simulink model "rtlsdr_rx_combinetwo"  (R2014b)
settings: Solver=ode45  StartTime=0.0  StopTime=inf  RelTol=1e-3
PreLoadFcn:
  | %%%%%%%%%%%%%%%%%%%%%%%%%%%%%%%%%%%%%%%%%%%%%%%%%%%%%%%%%%%%%%%%%%%%%%%%%%%
  | % check to see if Simulink library folder is missing from the MATLAB path %
  | %%%%%%%%%%%%%%%%%%%%%%%%%%%%%%%%%%%%%%%%%%%%%%%%%%%%%%%%%%%%%%%%%%%%%%%%%%%
  | if isempty(strfind(path, 'rtlsdr_book_library'))
  | 
  |     % create error window
  |     fig_error = figure(...
  |         'Name', 'Error: RTL-SDR Book Library',...
  |         'Toolbar','none',...
  |         'MenuBar','none',...
  |         'NumberTitle','off',...
  |         'Resize','off',...
  |         'WindowStyle','modal');
  |     fig_error.Position(3) = 600;
  |     fig_error.Position(4) = 150;
  |     fig_axes = axes(...
  |         'Parent',fig_error,...
  |         'Position',[0,0,1,1],...
  |         'visible','off');
  |     % error message
  |     t_title = text(.05,.8,...
  |         'MISSING DIRECTORIES',...
  |         'FontSize',11.5);
  |     t_body = text(.075,.6,...
  |         [{'Simulink cannot find the  \it{<root>}\rm / \it{rtlsdr\_book\_library}\rm  folder in the \it{MATLAB Path}\rm.'},...
  |         {'Please set the MATLAB path following the instructions given in Exercise 2.4.'}],...
  |         'FontSize',10.5);
  |     % buttons
  |     btn_path = uicontrol(...
  |         'Parent',fig_error,...
  |         'String','Set Path Now',...
  |         'FontSize',10,...
  |         'Callback', 'pathtool; close(fig_error);',...
  |         'Position', [fig_error.Position(3)/2-210, 30, 200, 30]);
  |     btn_abort = uicontrol(...
  |         'Parent',fig_error,...
  |         'String','No thanks',...
  |         'FontSize',10,...
  |         'Callback', 'close(fig_error); abort=1;',...
  |         'Position', [fig_error.Position(3)/2+10, 30, 200, 30]);
  | 
  |     % pause to allow user to interact with error box
  |     uiwait(fig_error);
  | 
  |     % abort simulation
  |     try
  |         if abort==1
  |             set_param(gcs, 'SimulationCommand', 'stop');
  |         end
  |     end
  | 
  |     % if user has set path, allow diagram to be updated
  |     if ~exist('abort','var')
  |         % create error window
  |         fig_update = figure(...
  |             'Name', 'Update Diagram',...
  |             'Toolbar','none',...
  |             'MenuBar','none',...
  |             'NumberTitle','off',...
  |             'Resize','off');
  |         fig_update.Position(3) = 400;
  |         fig_update.Position(4) = 120;
  |         fig_axes = axes(...
  |             'Parent',fig_update,...
  |             'Position',[0,0,1,1],...
  |             'visible','off');
  |         % instruction message
  |         t_body = text(.075,.7,...
  |             'Once you have set the path, update the block diagram',...
  |             'FontSize',10.5);
  |         % button
  |         btn_update = uicontrol(...
  |             'Parent',fig_update,...
  |             'String','Update Block Diagram',...
  |             'FontSize',10,...
  |             'Callback', 'set_param(gcs,''SimulationCommand'',''update''); close(gcf)',...
  |             'Position', [fig_update.Position(3)/2-100, 30, 200, 30]);
  |     end
  | 
  |     % clear error components
  |     clear('fig_error','fig_update','fig_axes','t_title','t_body','btn_path','btn_abort','btn_update','abort');
  | 
  | end
  | %%%%%%%%%%%%%%%%%%%%%%%%%%%%%%%%%%%%%%%%%%%%%%%%%%%%%%%%%%%%%%%%%%%%%%%%%%%
  | 
  | 
  | frm_size=4096;
  | rtlsdr_fs = 2.8e6;
StartFcn:
  | frm_size=4096;
  | rtlsdr_fs = 2.8e6;
undefined symbols (not defined in the file): Radix, set
libraries: rtlsdr_book_library x3, dspspect3 x2, sdrrlib x2, simulink x1
CloseFcn:
  | closefcn_model;
Description:
  | Software, Simulation Examples and Design Exercises Licence Agreement
  | 
  | This license agreement refers to the simulation examples, design exercises and files,
  | and associated software MATLAB and Simulink resources that accompany the book:
  | 
  |      Title: Software Defined Radio using MATLAB & Simulink and the RTL-SDR
  |      Published by Strathclyde Academic Media, 2015
  |      Authored by Robert W. Stewart, Kenneth W. Barlee, Dale S.W. Atkinson,
  |      and Louise H. Crockett
  | 
  | and made available as a download from, www.desktopSDR.com or variously acquired
  | by other means such as via USB storage, cloud storage, disk or any other electronic
  | or optical or magnetic storage mechanism. These files and associated software may
  | be used subject to the terms of agreement of the conditions below:
  | 
  |     Copyright © 2015 Robert W. Stewart, Kenneth W. Barlee, Dale S.W. Atkinson,
  |     and Louise H. Crockett
  |     All rights reserved.
  | 
  | Redistribution and use in source and binary forms, with or without modification, are
  | permitted provided that the following conditions are met:
  | 
  |    1.  Redistributions of source code must retain the above copyright notice, this list of
  |         conditions and the following disclaimer.
  | 
  |    2.  Redistributions in binary form must reproduce the above copyright notice, this
  |         list of conditions and the following disclaimer in the documentation and/or other
  |         materials provided with the distribution.
  | 
  |    3.  Neither the name of the copyright holder nor the names of its contributors may
  |         be used to endorse or promote products derived from this software without
  |         specific prior written permission.
  | 
  |    4.  In all cases, the software is, and all modifications and derivatives of the
  |         software shall be, licensed to you solely for use in conjunction with The
  |         MathWorks, Inc. products and service offerings.
  | 
  | THIS SOFTWARE IS PROVIDED BY THE COPYRIGHT HOLDERS AND CONTRIBUTORS
  | "AS IS" AND ANY EXPRESS OR IMPLIED WARRANTIES, INCLUDING, BUT NOT LIMITED
  | TO, THE IMPLIED WARRANTIES OF MERCHANTABILITY AND FITNESS FOR A
  | PARTICULAR PURPOSE ARE DISCLAIMED. IN NO EVENT SHALL THE COPYRIGHT
  | HOLDER OR CONTRIBUTORS BE LIABLE FOR ANY DIRECT, INDIRECT, INCIDENTAL,
  | SPECIAL, EXEMPLARY, OR CONSEQUENTIAL DAMAGES (INCLUDING, BUT NOT
  | LIMITED TO, PROCUREMENT OF SUBSTITUTE GOODS OR SERVICES; LOSS OF USE,
  | DATA, OR PROFITS; OR BUSINESS INTERRUPTION) HOWEVER CAUSED AND ON ANY
  | THEORY OF LIABILITY, WHETHER IN CONTRACT, STRICT LIABILITY, OR TORT
  | (INCLUDING NEGLIGENCE OR OTHERWISE) ARISING IN ANY WAY OUT OF THE USE
  | OF THIS SOFTWARE, EVEN IF ADVISED OF THE POSSIBILITY OF SUCH DAMAGE.
  | 
  | 
  | Audio Tracks used in Simulations Examples and Design Exercises
  | 
  | The music and vocal files used within the Examples files and software within the book
  | were variously written, arranged, performed, recorded and produced by Garrey Rice,
  | Adam Struth, Jamie Struth, Iain Thistlethwaite and also Marshall Craigmyle who
  | collectively, and individually where appropriate, assert and retain all of their copyright,
  | performance and artistic rights. Permission to use and reproduce this music is
  | granted for all purposes associated with MATLAB and Simulink software and the
  | simulation examples and design exercises files that accompany this book. Requests to
  | use the music for any other purpose should be directed to: info@desktopSDR.com.
  | For information on music track names, full credits, and links to the musicians please
  | refer to www.desktopSDR.com/more/audio.
settings Model: Creator=desktopSDR Team  LastModifiedBy=desktopSDR Team
settings DataIOCC: LimitDataPoints=off  SignalLoggingSaveFormat=ModelDataLogs  SaveOutput=off  SignalLogging=off  SaveTime=off
settings OptimizationCC: EfficientMapNaN2IntZero=off
settings DebuggingCC: UnderspecifiedInitializationDetection=Classic  MergeDetectMultiDrivingBlocksExec=none  MultiTaskDSMMsg=warning  MultiTaskCondExecSysMsg=none
settings HardwareCC: TargetLongLongMode=on  TargetIntDivRoundTo=Zero  TargetEndianess=LittleEndian  TargetHWDeviceType=MATLAB Host  ProdEqTarget=off
settings RTWCC: IncludeERTFirstTime=on
settings CodeAppCC: MaxIdLength=128
settings GRTTargetCC: CombineOutputUpdateFcns=off  GRTInterface=on

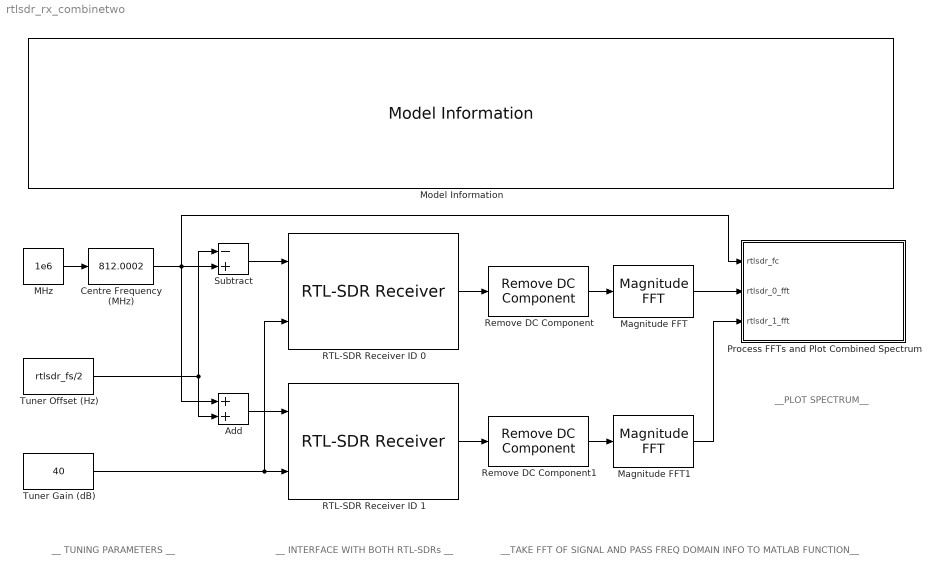
== system rtlsdr_rx_combinetwo ==
  note: __ TUNING PARAMETERS __
  note: __ INTERFACE WITH BOTH RTL-SDRs __
  note: __PLOT SPECTRUM__
  note: __TAKE FFT OF SIGNAL AND PASS FREQ DOMAIN INFO TO MATLAB FUNCTION__
  Add : Sum
  Centre Frequency (MHz) : simulink/Math Operations/Slider Gain  low=25  gain=812.0002  high=1750  mask(Slider Gain){}
      mask init:
      | open_system(gcb,'OpenFcn')
      mask Display:
      | % This is a new mask on top of the base mask.
      | % Use "View base mask" link below to see the base mask.
      | disp(num2str(get_param([gcb],'Gain')))
  MHz : Constant  Value=1e6
  Magnitude FFT : dspspect3/Magnitude FFT  mag_or_magsq=Magnitude  FFTImplementation=Radix-2  fftLenInherit=off  fftsize=1024  WrapInput=on
  Magnitude FFT1 : dspspect3/Magnitude FFT  mag_or_magsq=Magnitude  FFTImplementation=Radix-2  fftLenInherit=off  fftsize=1024  WrapInput=on
  Model Information : rtlsdr_book_library/Additional Tools/Model Information/Model Information
  Process FFTs and Plot Combined Spectrum : MATLAB Function  StopFcn=set(0,'DefaultFigureCloseRequestFcn','h_fig');  TreatAsAtomicUnit=on
  RTL-SDR Receiver ID 0 : sdrrlib/RTL-SDR Receiver  SourceLibraryInfo="This block requires <a href=\"http://www.mathworks.com/hardware-support/rtl-sdr.html\">Communications System Toolbox Support Package for RTL-SDR Radio</a>"  sobjType=sdrr.internal.SDRRTLReceiverSL  IPAddress=0  dataUDPPort=-1  ctrlUDPPort=-1  subDeviceList=nosubdev  sdrBlockType=SDRBlockTypeSLT.SDRRxBlock  requester=UNUSED_BY_SFCN  sdrExecutionMode=SDRExecutionModeSLT.ExecModeHW  LostSamplesOutputPort=off  OutputDataType=single  FrameLength=4096  EnableBurstMode=off  NumFramesInBurst=20  BypassUserLogic=off  DecimatorSelect=DDC decimator  SourceSelect=RF data  SineAmplitude=16000  EnableInternalClock=off  BypassIQBalance=off  CenterFrequency=102.5e6  IFBandwidth=40e6  ADCRateSource=Dialog  ADCRate=rtlsdr_fs  CenterFrequencySource=Input port  GainSource=Input port  IntermediateFrequency=0  Gain=0  DecimationFactorSource=Dialog  DecimationFactor=512  RFFrequencyIsTunable=logical(1)  SampleTime=(4096)/(rtlsdr_fs)  IFBandwidthSource=Dialog  SineFrequency=30000  BypassDCBlockingFilter=off  IntermediateFrequencySource=Dialog  IQBalanceCoefficients=64  SkipAllHardwareResetAndInitialization=off  EnableIQCalibrationTable=on  CacheIQCalibrationTable=off  EnableOffsetTuning=off  EnableRTLAGC=off  EnableTestMode=off  EnableTunerAGC=off  FrequencyCorrectionSource=Dialog  FrequencyCorrection=0  NumMLBuffers=128  NumUSBBuffers=16  LatencyOutputPort=off  RTLCrystalFrequency=28800000  TunerCrystalFrequency=28800000
  RTL-SDR Receiver ID 1 : sdrrlib/RTL-SDR Receiver  SourceLibraryInfo="This block requires <a href=\"http://www.mathworks.com/hardware-support/rtl-sdr.html\">Communications System Toolbox Support Package for RTL-SDR Radio</a>"  sobjType=sdrr.internal.SDRRTLReceiverSL  IPAddress=1  dataUDPPort=-1  ctrlUDPPort=-1  subDeviceList=nosubdev  sdrBlockType=SDRBlockTypeSLT.SDRRxBlock  requester=UNUSED_BY_SFCN  sdrExecutionMode=SDRExecutionModeSLT.ExecModeHW  LostSamplesOutputPort=off  OutputDataType=single  FrameLength=4096  EnableBurstMode=off  NumFramesInBurst=20  BypassUserLogic=off  DecimatorSelect=DDC decimator  SourceSelect=RF data  SineAmplitude=16000  EnableInternalClock=off  BypassIQBalance=off  CenterFrequency=102.5e6  IFBandwidth=40e6  ADCRateSource=Dialog  ADCRate=rtlsdr_fs  CenterFrequencySource=Input port  GainSource=Input port  IntermediateFrequency=0  Gain=0  DecimationFactorSource=Dialog  DecimationFactor=512  RFFrequencyIsTunable=logical(1)  SampleTime=(4096)/(rtlsdr_fs)  IFBandwidthSource=Dialog  SineFrequency=30000  BypassDCBlockingFilter=off  IntermediateFrequencySource=Dialog  IQBalanceCoefficients=64  SkipAllHardwareResetAndInitialization=off  EnableIQCalibrationTable=on  CacheIQCalibrationTable=off  EnableOffsetTuning=off  EnableRTLAGC=off  EnableTestMode=off  EnableTunerAGC=off  FrequencyCorrectionSource=Dialog  FrequencyCorrection=0  NumMLBuffers=128  NumUSBBuffers=16  LatencyOutputPort=off  RTLCrystalFrequency=28800000  TunerCrystalFrequency=28800000
  Remove DC Component : rtlsdr_book_library/Additional Tools/Remove DC Component
  Remove DC Component1 : rtlsdr_book_library/Additional Tools/Remove DC Component
  Subtract : Sum  Inputs=-+
  Tuner Gain (dB) : Constant  Value=40
  Tuner Offset (Hz) : Constant  Value=rtlsdr_fs/2
  wires:
  Subtract/1 -> RTL-SDR Receiver ID 0/1
  Tuner Offset (Hz)/1 -> Add/2, Subtract/1
  Tuner Gain (dB)/1 -> RTL-SDR Receiver ID 1/2, RTL-SDR Receiver ID 0/2
  Add/1 -> RTL-SDR Receiver ID 1/1
  Magnitude FFT/1 -> Process FFTs and Plot Combined Spectrum/2(rtlsdr_0_fft)
  Magnitude FFT1/1 -> Process FFTs and Plot Combined Spectrum/3(rtlsdr_1_fft)
  Centre Frequency (MHz)/1 -> Process FFTs and Plot Combined Spectrum/1(rtlsdr_fc), Add/1, Subtract/2
  MHz/1 -> Centre Frequency (MHz)/1
  RTL-SDR Receiver ID 0/1 -> Remove DC Component/1
  RTL-SDR Receiver ID 1/1 -> Remove DC Component1/1
  Remove DC Component/1 -> Magnitude FFT/1
  Remove DC Component1/1 -> Magnitude FFT1/1

== matlab function rtlsdr_rx_combinetwo/Process FFTs and Plot Combined Spectrum ==
  data: rtlsdr_fc input; rtlsdr_0_fft input; rtlsdr_1_fft input
%% Combining Two RTL-SDR Signals: Process FFT Data and Plot
% This function is used to process two fft matricies (from two RTL-SDRs),
% combine and plot the data in a figure window customised to look like a
% spectrum analyzer

function spectrum(rtlsdr_fc,rtlsdr_0_fft,rtlsdr_1_fft)

%% FUNCTION SETUP

% functions that cannot be compiled
coder.extrinsic('text');
coder.extrinsic('get');
coder.extrinsic('bdroot');
coder.extrinsic('eval');
coder.extrinsic('set_param');

% process inputs
assert(rtlsdr_fc >= 24e6);                          % limit range of centre frequnecy
assert(rtlsdr_fc <= 1700e6);                        % (required as the centre freq is a dynamic variable)
fft_len = length(rtlsdr_1_fft);                     % find size of ffts
rtlsdr_fc = rtlsdr_fc/1e6;                          % MHz downconvert
rtlsdr_fs = 2.8e6;                                  % sampling rate of RTL-SDR, must match model


%% CREATE FIGURE WINDOW
persistent h_fig
if isempty(h_fig)
    
    % find screen size
    scnsize = [0 0 0 0];
    scnsize = get(0,'ScreenSize');
    
    fig_width = 1200;
    fig_height = 350;
    fig_pos = [(scnsize(3)-fig_width)/2,(scnsize(4)-fig_height)/2,fig_width,fig_height];
    
    % create figure, centre on screen
    h_fig = figure(...
        'Name','Spectrum Analyzer - Data From Two RTL-SDRs',...
        'numbertitle', 'off',...
        'toolBar','none',...
        'CloseRequestFcn','closereq',...
        'Position',fig_pos);    
end
% colours
persistent line_blue window_grey axes_grey plot_white
if isempty(line_blue)
    line_blue = [0.0000 0.4470 0.7410];     % spectrum analyzer blue
end
if isempty(window_grey)
    window_grey = [0.95 0.95 0.95];         % background light grey
end
if isempty(axes_grey)
    axes_grey = [0.1 0.1 0.1];              % dark grey for axes titles etc
end
if isempty(plot_white)
    plot_white = [1 1 1];                   % white for plot background
end


%% MANIPULATE FFT DATA

% change to [+ve_0, -ve_0]
rtlsdr_0_reorder = 0:fft_len-1;
rtlsdr_0_reorder((fft_len/2)+1:end) = rtlsdr_0_fft(1:(fft_len/2));
rtlsdr_0_reorder(1:(fft_len/2)) = rtlsdr_0_fft((fft_len/2)+1:end);

% change to [+ve_1, -ve_1]
rtlsdr_1_reorder = 0:fft_len-1;
rtlsdr_1_reorder((fft_len/2)+1:end) = rtlsdr_1_fft(1:(fft_len/2));
rtlsdr_1_reorder(1:(fft_len/2)) = rtlsdr_1_fft((fft_len/2)+1:end);

% combine [+ve_0, -ve_0, +ve_1, -ve_1]
comb_fft = 0:(fft_len*2)-1;
comb_fft(fft_len+1:end) = rtlsdr_1_reorder;
comb_fft(1:fft_len) = rtlsdr_0_reorder;

%% PLOT DATA

% create xaxis
freq_bin = (rtlsdr_fs/1e6*2)/(fft_len*2);
x_freq = ((rtlsdr_fc)-fft_len*freq_bin)+freq_bin :freq_bin :((rtlsdr_fc)+fft_len*freq_bin);

% if figure is still open
if ishandle(h_fig)
    
    % format figure
    clf(h_fig);                                         % reset figure
    set(h_fig,'toolBar','none');
    set(h_fig,'name','Spectrum Analyzer - Data From Two RTL-SDRs','numbertitle','off');
    set(h_fig,'Renderer','painters');                   % change render mode to remove pixelation
    set(h_fig,'Color',window_grey);                     % window background
    
    %set(0,'CurrentFigure',h_fig);
    %set(0,'DefaultFigureCloseRequestFcn',@figclosereqfcn);
    
    % format axes
    h_axes = axes('Parent',h_fig);                      % create axes
    box(h_axes,'on');
    hold(h_axes,'on');
    grid(h_axes,'on');
    set(h_axes,'Color',plot_white);                     % plot background
    set(h_axes,'GridColor',axes_grey);                  % grid
    set(h_axes,'GridLineStyle','--');                   % dashed grid
    set(h_axes,'XColor',axes_grey);                     % xaxis colour
    set(h_axes,'YColor',axes_grey);                     % yaxis colour
    set(h_axes,'ZColor',axes_grey);                     % zaxis colour
    
    % calculate axes sizes
    fig_size = [0 0 0 0];                               % initialise to zero
    fig_size = get(h_fig,'position');                   % get figure size
    axis_x1 = 60/fig_size(3);                           % 60 pixels from left
    axis_y1 = 50/fig_size(4);                           % 50 pixels from bottom
    axis_x2 = (fig_size(3)-100)/fig_size(3);            % 100 pixels from right
    axis_y2 = (fig_size(4)-80)/fig_size(4);             % 80 pixels from top
    set(h_axes,'Position',[axis_x1 axis_y1 axis_x2 axis_y2]);
    
    % plot data
    plot(h_axes,x_freq',10*log10((comb_fft.^2)/50),'Color',line_blue,'linewidth',1.5);
    
    % limit plot display
    ylim(h_axes,[-60,30]);
    xlim(h_axes,[min(x_freq),max(x_freq)]);
    
    % axes labels
    title_x1 = min(x_freq)+((rtlsdr_fs/2)/1e6)-450/fig_size(3);            % centred at 25% of x
    title_x2 = min(x_freq)+(rtlsdr_fs/1e6)-30/fig_size(3);                 % centred at 50% of x
    title_x3 = min(x_freq)+((rtlsdr_fs/2+rtlsdr_fs)/1e6)-450/fig_size(3);  % centred at 75% of x
    title_y = 35-1.1/350*fig_size(4);                                      % in gap above axis
    title_rtlsdr0 = 'RTL-SDR Radio ID 0';
    title_split = '||';
    title_rtlsdr1 = 'RTL-SDR Radio ID 1';
    text(title_x1,title_y,title_rtlsdr0,'FontSize',13,'Parent',h_axes);
    text(title_x2,title_y,title_split,'FontSize',13,'Parent',h_axes);
    text(title_x3,title_y,title_rtlsdr1,'FontSize',13,'Parent',h_axes);
    xlabel(h_axes,'Frequency (MHz)','Color',axes_grey);
    ylabel(h_axes,'Power Ratio (dBm)  [relative to 50 \Omega load]','Color',axes_grey);
    
else
    
    % figure is closed, end simulation
    set_param(bdroot, 'SimulationCommand', 'stop');
    disp('');
    disp([bdroot,': Simulation terminated because the']);
    disp('spectrum analyzer figure window has been closed');
    disp('');
end

end
